simulink model "HeatConductionThroughIronRodSegmented"  (R2024b)
settings: Solver=VariableStepAuto  StartTime=0.0  StopTime=2500  MaxStep=100  RelTol=1e-3  AbsTol=1e-3  EnableMultiTasking=on
PreLoadFcn:
  | if ~exist('D', 'var')            D= 0.025;         end % [m]
  | if ~exist('L', 'var')            L= 0.2;           end % [m]
  | if ~exist('A', 'var')            A= pi*D^2/4;      end % [m^2]
  | if ~exist('A_cyl', 'var')        A_cyl= pi*D*L;    end % [m^2]
  | if ~exist('k', 'var')            k= 80.2;          end % [W/(K*m)]
  | if ~exist('h', 'var')            h= 32.1;          end % [W/(K*m)]
  | if ~exist('m', 'var')            m= 7800*A*L;      end % [kg]
  | if ~exist('c', 'var')            c= 447;           end % [J/kg/K]
  | if ~exist('T_air', 'var')        T_air= 20;        end % [degC]
  | if ~exist('T_base', 'var')       T_base= 100;      end % [degC]
  | if ~exist('T_init', 'var')       T_init= 20;       end % [degC]
  | if ~exist('num_segments', 'var') num_segments= 9; end % [degC]
undefined symbols (not defined in the file): A_cyl, L, m, num_segments, T_init
libraries: fl_lib x45, nesl_utility x7
Description:
  | Heat Conduction Through Iron Rod Using Segmented Model
settings Model: Creator=The MathWorks, Inc.  LastModifiedBy=The MathWorks, Inc.
settings SolverCC: AutoScaleAbsTol=off  AlgebraicLoopSolver=TrustRegion
settings DataIOCC: LimitDataPoints=on  SaveFormat=Array  ReturnWorkspaceOutputs=off  TimeSaveName=tout_segmented_mass_model  OutputSaveName=yout_segmented_mass_model
settings OptimizationCC: LifeSpan=inf
settings DebuggingCC: SolverPrmCheckMsg=warning  UnconnectedInputMsg=warning  UnconnectedOutputMsg=warning  UnconnectedLineMsg=warning  AllowSymbolicDim=off  PregeneratedLibrarySubsystemCodeDiagnostic=none  SFUnexpectedBacktrackingDiag=warning  SFNoUnconditionalDefaultTransitionDiag=warning  SFExecutionAtInitializationDiag=none  ArithmeticOperatorsInVariantConditions=warning
settings HardwareCC: ProdBitPerPointer=32  ProdBitPerSizeT=32  ProdBitPerPtrDiffT=32  ProdLargestAtomicFloat=None  ProdIntDivRoundTo=Undefined  ProdEndianess=Unspecified  ProdWordSize=32  ProdHWDeviceType=32-bit Generic
settings ModelReferenceCC: EnableRefExpFcnMdlSchedulingChecks=on  PropagateSignalLabelsOutOfModel=off
settings SFSimCC: SimUseLocalCustomCode=off  CustomCodeUndefinedFunction=UseInterfaceOnly
settings RTWCC: RTWUseLocalCustomCode=off  GPUComputeCapability=3.5  DLArmComputeVersion=19.05
settings CodeAppCC: StateflowObjectComments=on
settings GRTTargetCC: TargetLangStandard=C89/C90 (ANSI)
settings ConfigComp: CovMetricSettings=dw  CovSaveCumulativeToWorkspaceVar=on  CovSaveSingleToWorkspaceVar=on  CovExternalEMLEnable=off  CovSFcnEnable=off
settings SimscapeCC: SimscapeLogType=all  SimscapeLogSimulationStatistics=on  SimscapeLogName=simlog_HeatConductionThroughIronRodSegmented  SimscapeLogDataHistory=10000

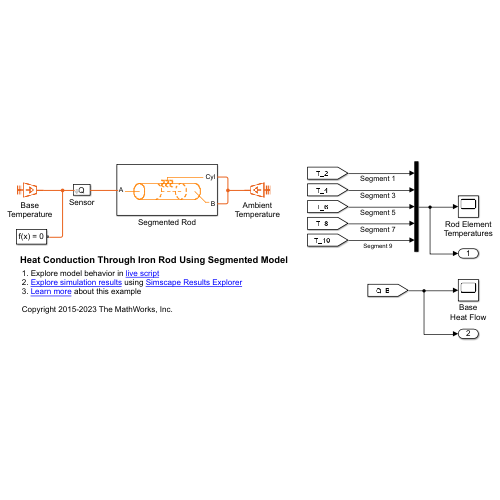
[thumbnail: Simulink's stored preview of the top-level diagram]
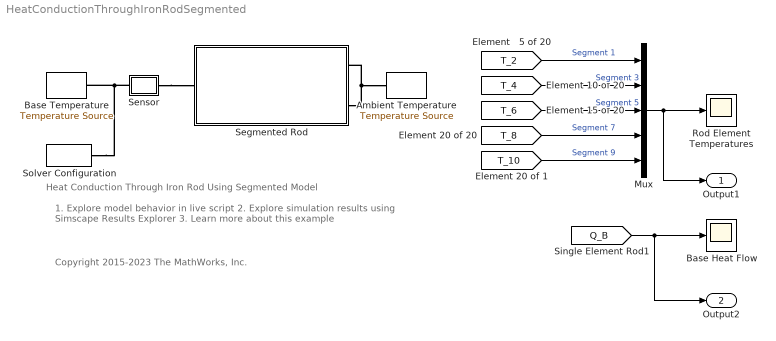
== system HeatConductionThroughIronRodSegmented ==
  note: Heat Conduction Through Iron Rod Using Segmented Model
  note: 1. Explore model behavior in live script
      | 2. Explore simulation results using Simscape Results Explorer
      | 3. Learn more about this example
  note: Copyright 2015-2023 The MathWorks, Inc.
  Ambient Temperature : fl_lib/Thermal/Thermal Sources/Temperature Source  temperature=T_air degC
  Base Heat Flow : Scope
  Base Temperature : fl_lib/Thermal/Thermal Sources/Temperature Source  temperature=T_base degC
  Mux : Mux  Inputs=5
  Rod Element Temperatures : Scope
  Segmented Rod : Subsystem  Tag=PublishSubsystem
      mask Display:
      | color('orange');
      | 
      | % Plot cylinder
      | plot([1,3],[1,1])
      | plot([1,3],[2,2])
      | plot(0.2*cos(0:2*pi/500:2*pi)+1,0.5*sin(0:2*pi/500:2*pi)+1.5)
      | plot(0.2*cos(-pi/2:2*pi/500:pi/2)+3,0.5*sin(-pi/2:2*pi/500:pi/2)+1.5)
      | 
      | % Plot Segmentation
      | plot(0.2*cos(0:2*pi/500:2*pi/16)+2.5,0.5*sin(0:2*pi/500:2*pi/16)+1.5)
      | plot(0.2*cos(2*2*pi/16:2*pi/500:3*2*pi/16)+2.5,0.5*sin(2*2*pi/16:2*pi/500:3*2*pi/16)+1.5)
      | plot(0.2*cos(4*2*pi/16:2*pi/500:5*2*pi/16)+2.5,0.5*sin(4*2*pi/16:2*pi/500:5*2*pi/16)+1.5)
      | plot(0.2*cos(6*2*pi/16:2*pi/500:7*2*pi/16)+2.5,0.5*sin(6*2*pi/16:2*pi/500:7*2*pi/16)+1.5)
      | plot(0.2*cos(8*2*pi/16:2*pi/500:9*2*pi/16)+2.5,0.5*sin(8*2*pi/16:2*pi/500:9*2*pi/16)+1.5)
      | plot(0.2*cos(10*2*pi/16:2*pi/500:11*2*pi/16)+2.5,0.5*sin(10*2*pi/16:2*pi/500:11*2*pi/16)+1.5)
      | plot(0.2*cos(12*2*pi/16:2*pi/500:13*2*pi/16)+2.5,0.5*sin(12*2*pi/16:2*pi/500:13*2*pi/16)+1.5)
      | plot(0.2*cos(14*2*pi/16:2*pi/500:15*2*pi/16)+2.5,0.5*sin(14*2*pi/16:2*pi/500:15*2*pi/16)+1.5)
      | 
      | plot(0.2*cos(0:2*pi/500:2*pi/16)+1.6,0.5*sin(0:2*pi/500:2*pi/16)+1.5)
      | plot(0.2*cos(2*2*pi/16:2*pi/500:3*2*pi/16)+1.6,0.5*sin(2*2*pi/16:2*pi/500:3*2*pi/16)+1.5)
      | plot(0.2*cos(12*2*pi/16:2*pi/500:13*2*pi/16)+1.6,0.5*sin(12*2*pi/16:2*pi/500:13*2*pi/16)+1.5)
      | plot(0.2*cos(14*2*pi/16:2*pi/500:15*2*pi/16)+1.6,0.5*sin(14*2*pi/16:2*pi/500:15*2*pi/16)+1.5)
      | 
      | plot([1.8 1.9],[1.5 1.5])
      | plot([2 2.1],[1.5 1.5])
      | plot([2.2 2.3],[1.5 1.5])
      | plot([2.4 2.5],[1.5 1.5])
      | 
      | % Heat Port
      | plot([1.8 2.2],[2.2 2.2])
      | plot([0.1*cos(-pi/2:0.1:pi/2)+1.8],[0.1*sin(-pi/2:0.1:pi/2)+2.1])
      | plot([0.1*cos(pi/2:0.1:3*pi/2)+1.9],[0.1*sin(pi/2:0.1:3*pi/2)+1.9])
      | plot([0.1*cos(-pi/2:0.1:pi/2)+1.95],[0.1*sin(-pi/2:0.1:pi/2)+2.1])
      | plot([0.1*cos(pi/2:0.1:3*pi/2)+2.05],[0.1*sin(pi/2:0.1:3*pi/2)+1.9])
      | plot([0.1*cos(-pi/2:0.1:pi/2)+2.1],[0.1*sin(-pi/2:0.1:pi/2)+2.1])
      | plot([0.1*cos(pi/2:0.1:3*pi/2)+2.2],[0.1*sin(pi/2:0.1:3*pi/2)+1.9])
      | 
      | % Connecting lines
      | plot([2 3.3],[2.4,2.4])
      | plot([2 2],[2.2 2.4])
      | plot([0.5 1],[1.5 1.5])
      | plot([3.4 3.5],[0.8 0.8])
      | plot([3,3.4],[1.5 0.8])
      | % Scaling
      | color('white')
      | plot(0.2,0)
      | plot(3.8,3.2)
  Sensor : Subsystem
      mask Display: fprintf('Q')
  Solver Configuration : nesl_utility/Solver Configuration  PhysicalDomain=network_engine_domain  SubClassName=solver  LeftPortType=input  RightPortType=generic  Tones=[]  Harmonics=[]  SimulateNoise=off  Profile=off  UseLocalSampling=off  EnableSwitchedLinearOptims=on  FrequencyDomain=off  UseCCode=off  RelTol=0.001  AbsTol=1e-06  MinStep=1e-09  ToWorkspace=off  RevertToSquareIcSolve=off  NumHomotopyIterations=100  PhasorMode=off  PhasorModeNumHarmonics=1  ConsistencySolver=NEWTON_XTOL_AFTER_FTOL  IndexReductionMethod=DerivativeReplacement  DoDC=off  ResidualTolerance=1e-9  ConsistencyTolSource=GLOBAL  ConsistencyAbsTol=0.001  ConsistencyRelTol=0.001  ConsistencyTolFactor=0.001  UseLocalSolver=off  LocalSolverChoice=NE_BACKWARD_EULER_ADVANCER  ResolveIndetEquations=on  FunctionEvalNumThread=1  LocalSolverSampleTime=.001  DoFixedCost=off  MaxNonlinIter=3  MaxModeIter=2  ComputeImpulses=off  ImpulseIterations=2  LinearAlgebra=auto  LinearAlgebraNumThread=0  EquationFormulation=NE_TIME_EF  DelaysMemoryBudget=1024  AutomaticFiltering=on  FilteringTimeConstant=0.001  PartitionStorageMethod=AS_NEEDED  PartitionMemoryBudget=1024  PartitionMethod=FAST  MultibodyUseLocalSolver=off  MultibodyLocalSolverChoice=ODE1  MultibodyLocalSolverSampleTime=0.001
  Output1 : Outport
  Output2 : Outport  Port=2
  wires:
  Mux/1 -> Rod Element Temperatures/1, Output1/1
  [T_6] -> Mux/3  "Segment 5"
  [T_2] -> Mux/1  "Segment 1"
  [T_4] -> Mux/2  "Segment 3"
  [T_8] -> Mux/4  "Segment 7"
  [Q_B] -> Output2/1, Base Heat Flow/1
  [T_10] -> Mux/5  "Segment 9"
  connections:
  Segmented Rod/RConn2 -- Ambient Temperature/LConn1 -- Segmented Rod/RConn1
  Sensor/LConn1 -- Solver Configuration/RConn1 -- Base Temperature/LConn1
  Sensor/RConn1 -- Segmented Rod/LConn1

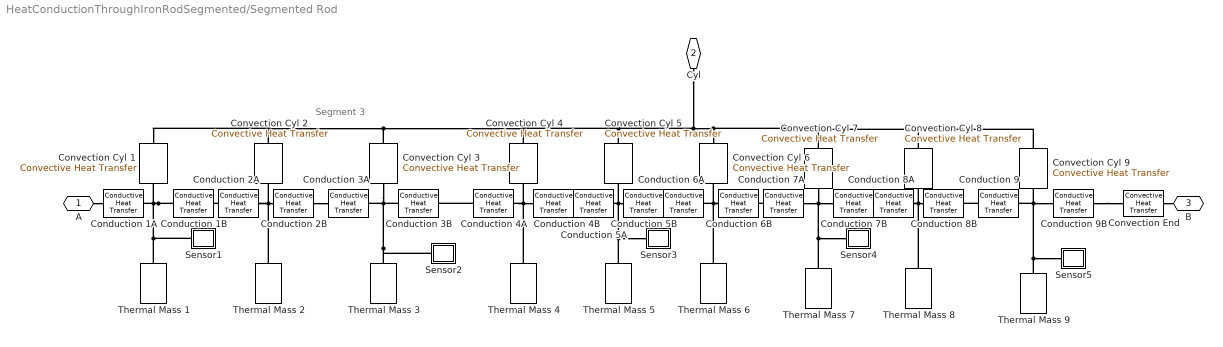
== system HeatConductionThroughIronRodSegmented/Segmented Rod ==
  note: Segment 3
  Conduction 1A : fl_lib/Thermal/Thermal Elements/Conductive Heat Transfer  thermal_type=foundation.enum.ConstantVariableTabulated.Constant  wall_geometry=foundation.enum.ConductionWallGeometry.Planar  area=A m^2  thickness=L/(2*num_segments) m  d_in=0.05 m  d_out=0.1 m  L=1 m  th_cond_min=10 W/(K*m)  th_cond=k W/m/K  th_cond_TLU=[413, 401, 392, 383, 371, 357, 342] W/(K*m)  temp_TLU=[200, 273, 400, 600, 800, 1000, 1200] K  T_specify=off  T_priority=High  T=0 K  T_nominal_specify=off  T_nominal_value=1  T_nominal_unit=K  Q_specify=off  Q_priority=High  Q=0 J/s  Q_nominal_specify=off  Q_nominal_value=1  Q_nominal_unit=J/s
  Conduction 1B : fl_lib/Thermal/Thermal Elements/Conductive Heat Transfer  thermal_type=foundation.enum.ConstantVariableTabulated.Constant  wall_geometry=foundation.enum.ConductionWallGeometry.Planar  area=A m^2  thickness=L/(2*num_segments) m  d_in=0.05 m  d_out=0.1 m  L=1 m  th_cond_min=10 W/(K*m)  th_cond=k W/m/K  th_cond_TLU=[413, 401, 392, 383, 371, 357, 342] W/(K*m)  temp_TLU=[200, 273, 400, 600, 800, 1000, 1200] K  T_specify=off  T_priority=High  T=0 K  T_nominal_specify=off  T_nominal_value=1  T_nominal_unit=K  Q_specify=off  Q_priority=High  Q=0 J/s  Q_nominal_specify=off  Q_nominal_value=1  Q_nominal_unit=J/s
  Conduction 2A : fl_lib/Thermal/Thermal Elements/Conductive Heat Transfer  thermal_type=foundation.enum.ConstantVariableTabulated.Constant  wall_geometry=foundation.enum.ConductionWallGeometry.Planar  area=A m^2  thickness=L/(2*num_segments) m  d_in=0.05 m  d_out=0.1 m  L=1 m  th_cond_min=10 W/(K*m)  th_cond=k W/m/K  th_cond_TLU=[413, 401, 392, 383, 371, 357, 342] W/(K*m)  temp_TLU=[200, 273, 400, 600, 800, 1000, 1200] K  T_specify=off  T_priority=High  T=0 K  T_nominal_specify=off  T_nominal_value=1  T_nominal_unit=K  Q_specify=off  Q_priority=High  Q=0 J/s  Q_nominal_specify=off  Q_nominal_value=1  Q_nominal_unit=J/s
  Conduction 2B : fl_lib/Thermal/Thermal Elements/Conductive Heat Transfer  thermal_type=foundation.enum.ConstantVariableTabulated.Constant  wall_geometry=foundation.enum.ConductionWallGeometry.Planar  area=A m^2  thickness=L/(2*num_segments) m  d_in=0.05 m  d_out=0.1 m  L=1 m  th_cond_min=10 W/(K*m)  th_cond=k W/m/K  th_cond_TLU=[413, 401, 392, 383, 371, 357, 342] W/(K*m)  temp_TLU=[200, 273, 400, 600, 800, 1000, 1200] K  T_specify=off  T_priority=High  T=0 K  T_nominal_specify=off  T_nominal_value=1  T_nominal_unit=K  Q_specify=off  Q_priority=High  Q=0 J/s  Q_nominal_specify=off  Q_nominal_value=1  Q_nominal_unit=J/s
  Conduction 3A : fl_lib/Thermal/Thermal Elements/Conductive Heat Transfer  thermal_type=foundation.enum.ConstantVariableTabulated.Constant  wall_geometry=foundation.enum.ConductionWallGeometry.Planar  area=A m^2  thickness=L/(2*num_segments) m  d_in=0.05 m  d_out=0.1 m  L=1 m  th_cond_min=10 W/(K*m)  th_cond=k W/m/K  th_cond_TLU=[413, 401, 392, 383, 371, 357, 342] W/(K*m)  temp_TLU=[200, 273, 400, 600, 800, 1000, 1200] K  T_specify=off  T_priority=High  T=0 K  T_nominal_specify=off  T_nominal_value=1  T_nominal_unit=K  Q_specify=off  Q_priority=High  Q=0 J/s  Q_nominal_specify=off  Q_nominal_value=1  Q_nominal_unit=J/s
  Conduction 3B : fl_lib/Thermal/Thermal Elements/Conductive Heat Transfer  thermal_type=foundation.enum.ConstantVariableTabulated.Constant  wall_geometry=foundation.enum.ConductionWallGeometry.Planar  area=A m^2  thickness=L/(2*num_segments) m  d_in=0.05 m  d_out=0.1 m  L=1 m  th_cond_min=10 W/(K*m)  th_cond=k W/m/K  th_cond_TLU=[413, 401, 392, 383, 371, 357, 342] W/(K*m)  temp_TLU=[200, 273, 400, 600, 800, 1000, 1200] K  T_specify=off  T_priority=High  T=0 K  T_nominal_specify=off  T_nominal_value=1  T_nominal_unit=K  Q_specify=off  Q_priority=High  Q=0 J/s  Q_nominal_specify=off  Q_nominal_value=1  Q_nominal_unit=J/s
  Conduction 4A : fl_lib/Thermal/Thermal Elements/Conductive Heat Transfer  thermal_type=foundation.enum.ConstantVariableTabulated.Constant  wall_geometry=foundation.enum.ConductionWallGeometry.Planar  area=A m^2  thickness=L/(2*num_segments) m  d_in=0.05 m  d_out=0.1 m  L=1 m  th_cond_min=10 W/(K*m)  th_cond=k W/m/K  th_cond_TLU=[413, 401, 392, 383, 371, 357, 342] W/(K*m)  temp_TLU=[200, 273, 400, 600, 800, 1000, 1200] K  T_specify=off  T_priority=High  T=0 K  T_nominal_specify=off  T_nominal_value=1  T_nominal_unit=K  Q_specify=off  Q_priority=High  Q=0 J/s  Q_nominal_specify=off  Q_nominal_value=1  Q_nominal_unit=J/s
  Conduction 4B : fl_lib/Thermal/Thermal Elements/Conductive Heat Transfer  thermal_type=foundation.enum.ConstantVariableTabulated.Constant  wall_geometry=foundation.enum.ConductionWallGeometry.Planar  area=A m^2  thickness=L/(2*num_segments) m  d_in=0.05 m  d_out=0.1 m  L=1 m  th_cond_min=10 W/(K*m)  th_cond=k W/m/K  th_cond_TLU=[413, 401, 392, 383, 371, 357, 342] W/(K*m)  temp_TLU=[200, 273, 400, 600, 800, 1000, 1200] K  T_specify=off  T_priority=High  T=0 K  T_nominal_specify=off  T_nominal_value=1  T_nominal_unit=K  Q_specify=off  Q_priority=High  Q=0 J/s  Q_nominal_specify=off  Q_nominal_value=1  Q_nominal_unit=J/s
  Conduction 5A : fl_lib/Thermal/Thermal Elements/Conductive Heat Transfer  thermal_type=foundation.enum.ConstantVariableTabulated.Constant  wall_geometry=foundation.enum.ConductionWallGeometry.Planar  area=A m^2  thickness=L/(2*num_segments) m  d_in=0.05 m  d_out=0.1 m  L=1 m  th_cond_min=10 W/(K*m)  th_cond=k W/m/K  th_cond_TLU=[413, 401, 392, 383, 371, 357, 342] W/(K*m)  temp_TLU=[200, 273, 400, 600, 800, 1000, 1200] K  T_specify=off  T_priority=High  T=0 K  T_nominal_specify=off  T_nominal_value=1  T_nominal_unit=K  Q_specify=off  Q_priority=High  Q=0 J/s  Q_nominal_specify=off  Q_nominal_value=1  Q_nominal_unit=J/s
  Conduction 5B : fl_lib/Thermal/Thermal Elements/Conductive Heat Transfer  thermal_type=foundation.enum.ConstantVariableTabulated.Constant  wall_geometry=foundation.enum.ConductionWallGeometry.Planar  area=A m^2  thickness=L/(2*num_segments) m  d_in=0.05 m  d_out=0.1 m  L=1 m  th_cond_min=10 W/(K*m)  th_cond=k W/m/K  th_cond_TLU=[413, 401, 392, 383, 371, 357, 342] W/(K*m)  temp_TLU=[200, 273, 400, 600, 800, 1000, 1200] K  T_specify=off  T_priority=High  T=0 K  T_nominal_specify=off  T_nominal_value=1  T_nominal_unit=K  Q_specify=off  Q_priority=High  Q=0 J/s  Q_nominal_specify=off  Q_nominal_value=1  Q_nominal_unit=J/s
  Conduction 6A : fl_lib/Thermal/Thermal Elements/Conductive Heat Transfer  thermal_type=foundation.enum.ConstantVariableTabulated.Constant  wall_geometry=foundation.enum.ConductionWallGeometry.Planar  area=A m^2  thickness=L/(2*num_segments) m  d_in=0.05 m  d_out=0.1 m  L=1 m  th_cond_min=10 W/(K*m)  th_cond=k W/m/K  th_cond_TLU=[413, 401, 392, 383, 371, 357, 342] W/(K*m)  temp_TLU=[200, 273, 400, 600, 800, 1000, 1200] K  T_specify=off  T_priority=High  T=0 K  T_nominal_specify=off  T_nominal_value=1  T_nominal_unit=K  Q_specify=off  Q_priority=High  Q=0 J/s  Q_nominal_specify=off  Q_nominal_value=1  Q_nominal_unit=J/s
  Conduction 6B : fl_lib/Thermal/Thermal Elements/Conductive Heat Transfer  thermal_type=foundation.enum.ConstantVariableTabulated.Constant  wall_geometry=foundation.enum.ConductionWallGeometry.Planar  area=A m^2  thickness=L/(2*num_segments) m  d_in=0.05 m  d_out=0.1 m  L=1 m  th_cond_min=10 W/(K*m)  th_cond=k W/m/K  th_cond_TLU=[413, 401, 392, 383, 371, 357, 342] W/(K*m)  temp_TLU=[200, 273, 400, 600, 800, 1000, 1200] K  T_specify=off  T_priority=High  T=0 K  T_nominal_specify=off  T_nominal_value=1  T_nominal_unit=K  Q_specify=off  Q_priority=High  Q=0 J/s  Q_nominal_specify=off  Q_nominal_value=1  Q_nominal_unit=J/s
  Conduction 7A : fl_lib/Thermal/Thermal Elements/Conductive Heat Transfer  thermal_type=foundation.enum.ConstantVariableTabulated.Constant  wall_geometry=foundation.enum.ConductionWallGeometry.Planar  area=A m^2  thickness=L/(2*num_segments) m  d_in=0.05 m  d_out=0.1 m  L=1 m  th_cond_min=10 W/(K*m)  th_cond=k W/m/K  th_cond_TLU=[413, 401, 392, 383, 371, 357, 342] W/(K*m)  temp_TLU=[200, 273, 400, 600, 800, 1000, 1200] K  T_specify=off  T_priority=High  T=0 K  T_nominal_specify=off  T_nominal_value=1  T_nominal_unit=K  Q_specify=off  Q_priority=High  Q=0 J/s  Q_nominal_specify=off  Q_nominal_value=1  Q_nominal_unit=J/s
  Conduction 7B : fl_lib/Thermal/Thermal Elements/Conductive Heat Transfer  thermal_type=foundation.enum.ConstantVariableTabulated.Constant  wall_geometry=foundation.enum.ConductionWallGeometry.Planar  area=A m^2  thickness=L/(2*num_segments) m  d_in=0.05 m  d_out=0.1 m  L=1 m  th_cond_min=10 W/(K*m)  th_cond=k W/m/K  th_cond_TLU=[413, 401, 392, 383, 371, 357, 342] W/(K*m)  temp_TLU=[200, 273, 400, 600, 800, 1000, 1200] K  T_specify=off  T_priority=High  T=0 K  T_nominal_specify=off  T_nominal_value=1  T_nominal_unit=K  Q_specify=off  Q_priority=High  Q=0 J/s  Q_nominal_specify=off  Q_nominal_value=1  Q_nominal_unit=J/s
  Conduction 8A : fl_lib/Thermal/Thermal Elements/Conductive Heat Transfer  thermal_type=foundation.enum.ConstantVariableTabulated.Constant  wall_geometry=foundation.enum.ConductionWallGeometry.Planar  area=A m^2  thickness=L/(2*num_segments) m  d_in=0.05 m  d_out=0.1 m  L=1 m  th_cond_min=10 W/(K*m)  th_cond=k W/m/K  th_cond_TLU=[413, 401, 392, 383, 371, 357, 342] W/(K*m)  temp_TLU=[200, 273, 400, 600, 800, 1000, 1200] K  T_specify=off  T_priority=High  T=0 K  T_nominal_specify=off  T_nominal_value=1  T_nominal_unit=K  Q_specify=off  Q_priority=High  Q=0 J/s  Q_nominal_specify=off  Q_nominal_value=1  Q_nominal_unit=J/s
  Conduction 8B : fl_lib/Thermal/Thermal Elements/Conductive Heat Transfer  thermal_type=foundation.enum.ConstantVariableTabulated.Constant  wall_geometry=foundation.enum.ConductionWallGeometry.Planar  area=A m^2  thickness=L/(2*num_segments) m  d_in=0.05 m  d_out=0.1 m  L=1 m  th_cond_min=10 W/(K*m)  th_cond=k W/m/K  th_cond_TLU=[413, 401, 392, 383, 371, 357, 342] W/(K*m)  temp_TLU=[200, 273, 400, 600, 800, 1000, 1200] K  T_specify=off  T_priority=High  T=0 K  T_nominal_specify=off  T_nominal_value=1  T_nominal_unit=K  Q_specify=off  Q_priority=High  Q=0 J/s  Q_nominal_specify=off  Q_nominal_value=1  Q_nominal_unit=J/s
  Conduction 9 : fl_lib/Thermal/Thermal Elements/Conductive Heat Transfer  thermal_type=foundation.enum.ConstantVariableTabulated.Constant  wall_geometry=foundation.enum.ConductionWallGeometry.Planar  area=A m^2  thickness=L/(2*num_segments) m  d_in=0.05 m  d_out=0.1 m  L=1 m  th_cond_min=10 W/(K*m)  th_cond=k W/m/K  th_cond_TLU=[413, 401, 392, 383, 371, 357, 342] W/(K*m)  temp_TLU=[200, 273, 400, 600, 800, 1000, 1200] K  T_specify=off  T_priority=High  T=0 K  T_nominal_specify=off  T_nominal_value=1  T_nominal_unit=K  Q_specify=off  Q_priority=High  Q=0 J/s  Q_nominal_specify=off  Q_nominal_value=1  Q_nominal_unit=J/s
  Conduction 9B : fl_lib/Thermal/Thermal Elements/Conductive Heat Transfer  thermal_type=foundation.enum.ConstantVariableTabulated.Constant  wall_geometry=foundation.enum.ConductionWallGeometry.Planar  area=A m^2  thickness=L/(2*num_segments) m  d_in=0.05 m  d_out=0.1 m  L=1 m  th_cond_min=10 W/(K*m)  th_cond=k W/m/K  th_cond_TLU=[413, 401, 392, 383, 371, 357, 342] W/(K*m)  temp_TLU=[200, 273, 400, 600, 800, 1000, 1200] K  T_specify=off  T_priority=High  T=0 K  T_nominal_specify=off  T_nominal_value=1  T_nominal_unit=K  Q_specify=off  Q_priority=High  Q=0 J/s  Q_nominal_specify=off  Q_nominal_value=1  Q_nominal_unit=J/s
  Convection Cyl {1..9} (9 alike) : fl_lib/Thermal/Thermal Elements/Convective Heat Transfer  thermal_type=foundation.enum.constant_variable.constant  area=A_cyl/num_segments m^2  heat_tr_coeff=h W/m^2/K  min_heat_tr_coeff=1e-3 W/(K*m^2)  T_specify=off  T_priority=High  T=0 K  T_nominal_specify=off  T_nominal_value=1  T_nominal_unit=K  Q_specify=off  Q_priority=High  Q=0 J/s  Q_nominal_specify=off  Q_nominal_value=1  Q_nominal_unit=J/s
  Convection End : fl_lib/Thermal/Thermal Elements/Convective Heat Transfer  thermal_type=foundation.enum.constant_variable.constant  area=A m^2  heat_tr_coeff=h W/(m^2 * K)  min_heat_tr_coeff=1e-3 W/(K*m^2)  T_specify=off  T_priority=None  T=0 K  T_nominal_specify=off  T_nominal_value=1  T_nominal_unit=K  Q_specify=off  Q_priority=None  Q=0 W  Q_nominal_specify=off  Q_nominal_value=1  Q_nominal_unit=W
  Sensor1 : Subsystem
      mask Display: disp('T')
  Sensor2 : Subsystem
      mask Display: disp('T')
  Sensor3 : Subsystem
      mask Display: disp('T')
  Sensor4 : Subsystem
      mask Display: disp('T')
  Sensor5 : Subsystem
      mask Display: disp('T')
  Thermal Mass {1..9} (9 alike) : fl_lib/Thermal/Thermal Elements/Thermal Mass  mass_type=foundation.enum.constant_variable.constant  mass=m/num_segments kg  sp_heat=c J/kg/K  mass_min=1e-6 kg  num_ports=foundation.enum.numPorts2.one  m_specify=off  m_priority=High  m=1 kg  m_nominal_specify=off  m_nominal_value=1  m_nominal_unit=kg  T_specify=on  T_priority=High  T=T_init degC  T_nominal_specify=off  T_nominal_value=1  T_nominal_unit=K  Q_specify=off  Q_priority=None  Q=0 W  Q_nominal_specify=off  Q_nominal_value=1  Q_nominal_unit=W
  A : PMIOPort  Side=Left
  Cyl : PMIOPort  Port=2  Side=Right
  B : PMIOPort  Port=3  Side=Right
  connections:
  Conduction 5A/LConn1 -- Conduction 4B/RConn1
  Conduction 2B/RConn1 -- Conduction 3A/LConn1
  A/RConn1 -- Conduction 1A/LConn1
  Conduction 2A/LConn1 -- Conduction 1B/RConn1
  Conduction 4A/LConn1 -- Conduction 3B/RConn1
  Convection Cyl 5/LConn1 -- Thermal Mass 5/LConn1 -- Sensor3/LConn1 -- Conduction 5A/RConn1 -- Conduction 5B/LConn1
  Conduction 4B/LConn1 -- Thermal Mass 4/LConn1 -- Convection Cyl 4/LConn1 -- Conduction 4A/RConn1
  Thermal Mass 3/LConn1 -- Sensor2/LConn1 -- Conduction 3B/LConn1 -- Convection Cyl 3/LConn1 -- Conduction 3A/RConn1
  Conduction 2B/LConn1 -- Thermal Mass 2/LConn1 -- Conduction 2A/RConn1 -- Convection Cyl 2/LConn1
  Thermal Mass 1/LConn1 -- Sensor1/LConn1 -- Conduction 1B/LConn1 -- Conduction 1A/RConn1 -- Convection Cyl 1/LConn1
  Conduction 7B/RConn1 -- Conduction 8A/LConn1
  Conduction 5B/RConn1 -- Conduction 6A/LConn1
  Conduction 7A/LConn1 -- Conduction 6B/RConn1
  Conduction 6A/RConn1 -- Thermal Mass 6/LConn1 -- Convection Cyl 6/LConn1 -- Conduction 6B/LConn1
  Cyl/RConn1 -- Convection Cyl 5/RConn1 -- Convection Cyl 2/RConn1 -- Convection Cyl 1/RConn1 -- Convection Cyl 3/RConn1 -- Convection Cyl 4/RConn1 -- Convection Cyl 9/RConn1 -- Convection Cyl 8/RConn1 -- Convection Cyl 7/RConn1 -- Convection Cyl 6/RConn1
  Conduction 7A/RConn1 -- Sensor4/LConn1 -- Thermal Mass 7/LConn1 -- Conduction 7B/LConn1 -- Convection Cyl 7/LConn1
  Conduction 8B/LConn1 -- Thermal Mass 8/LConn1 -- Convection Cyl 8/LConn1 -- Conduction 8A/RConn1
  Conduction 9/RConn1 -- Thermal Mass 9/LConn1 -- Sensor5/LConn1 -- Convection Cyl 9/LConn1 -- Conduction 9B/LConn1
  Conduction 9/LConn1 -- Conduction 8B/RConn1
  Conduction 9B/RConn1 -- Convection End/LConn1
  Convection End/RConn1 -- B/RConn1

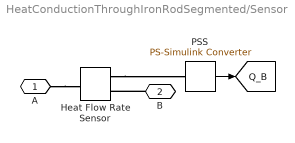
== system HeatConductionThroughIronRodSegmented/Sensor ==
  Heat Flow Rate Sensor : fl_lib/Thermal/Thermal Sensors/Heat Flow Rate Sensor
  PSS : nesl_utility/PS-Simulink Converter  PhysicalDomain=network_engine_domain  SubClassName=ps_output  LeftPortType=input  RightPortType=output  PseudoPeriodic=off  Frequencies=[]  VectorFormat=1-D array  Unit=W  AffineConversion=off
  A : PMIOPort  Side=Left
  B : PMIOPort  Port=2  Side=Right
  tag scope: Q_B=global
  wires:
  PSS/1 -> [Q_B]
  connections:
  A/RConn1 -- Heat Flow Rate Sensor/LConn1
  B/RConn1 -- Heat Flow Rate Sensor/RConn2
  Heat Flow Rate Sensor/RConn1 -- PSS/LConn1

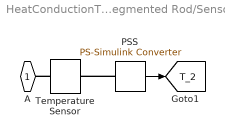
== system HeatConductionThroughIronRodSegmented/Segmented Rod/Sensor1 ==
  PSS : nesl_utility/PS-Simulink Converter  PhysicalDomain=network_engine_domain  SubClassName=ps_output  LeftPortType=input  RightPortType=output  PseudoPeriodic=off  Frequencies=[]  VectorFormat=1-D array  Unit=degC  AffineConversion=on
  Temperature Sensor : fl_lib/Thermal/Thermal Sensors/Temperature Sensor  temperature_measure=foundation.enum.MeasurementReference.absolute
      settings: InternalSimscapePortConfiguration="{\"Bottom\":[],\"Left\":[{\"id\":\"A\",\"label\":\"A\",\"type\":\"foundation.thermal.thermal\"}],\"Right\":[{\"id\":\"T\",\"label\":\"T\",\"type\":\"output\"}],\"Top\":[]}"
  A : PMIOPort  Side=Left
  tag scope: T_2=global
  wires:
  PSS/1 -> [T_2]
  connections:
  PSS/LConn1 -- Temperature Sensor/RConn1
  Temperature Sensor/LConn1 -- A/RConn1

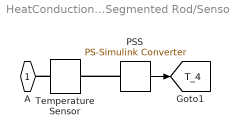
== system HeatConductionThroughIronRodSegmented/Segmented Rod/Sensor2 ==
  PSS : nesl_utility/PS-Simulink Converter  PhysicalDomain=network_engine_domain  SubClassName=ps_output  LeftPortType=input  RightPortType=output  PseudoPeriodic=off  Frequencies=[]  VectorFormat=1-D array  Unit=degC  AffineConversion=on
  Temperature Sensor : fl_lib/Thermal/Thermal Sensors/Temperature Sensor  temperature_measure=foundation.enum.MeasurementReference.absolute
      settings: InternalSimscapePortConfiguration="{\"Bottom\":[],\"Left\":[{\"id\":\"A\",\"label\":\"A\",\"type\":\"foundation.thermal.thermal\"}],\"Right\":[{\"id\":\"T\",\"label\":\"T\",\"type\":\"output\"}],\"Top\":[]}"
  A : PMIOPort  Side=Left
  tag scope: T_4=global
  wires:
  PSS/1 -> [T_4]
  connections:
  PSS/LConn1 -- Temperature Sensor/RConn1
  Temperature Sensor/LConn1 -- A/RConn1

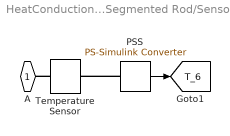
== system HeatConductionThroughIronRodSegmented/Segmented Rod/Sensor3 ==
  PSS : nesl_utility/PS-Simulink Converter  PhysicalDomain=network_engine_domain  SubClassName=ps_output  LeftPortType=input  RightPortType=output  PseudoPeriodic=off  Frequencies=[]  VectorFormat=1-D array  Unit=degC  AffineConversion=on
  Temperature Sensor : fl_lib/Thermal/Thermal Sensors/Temperature Sensor  temperature_measure=foundation.enum.MeasurementReference.absolute
      settings: InternalSimscapePortConfiguration="{\"Bottom\":[],\"Left\":[{\"id\":\"A\",\"label\":\"A\",\"type\":\"foundation.thermal.thermal\"}],\"Right\":[{\"id\":\"T\",\"label\":\"T\",\"type\":\"output\"}],\"Top\":[]}"
  A : PMIOPort  Side=Left
  tag scope: T_6=global
  wires:
  PSS/1 -> [T_6]
  connections:
  PSS/LConn1 -- Temperature Sensor/RConn1
  Temperature Sensor/LConn1 -- A/RConn1

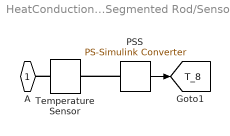
== system HeatConductionThroughIronRodSegmented/Segmented Rod/Sensor4 ==
  PSS : nesl_utility/PS-Simulink Converter  PhysicalDomain=network_engine_domain  SubClassName=ps_output  LeftPortType=input  RightPortType=output  PseudoPeriodic=off  Frequencies=[]  VectorFormat=1-D array  Unit=degC  AffineConversion=on
  Temperature Sensor : fl_lib/Thermal/Thermal Sensors/Temperature Sensor  temperature_measure=foundation.enum.MeasurementReference.absolute
      settings: InternalSimscapePortConfiguration="{\"Bottom\":[],\"Left\":[{\"id\":\"A\",\"label\":\"A\",\"type\":\"foundation.thermal.thermal\"}],\"Right\":[{\"id\":\"T\",\"label\":\"T\",\"type\":\"output\"}],\"Top\":[]}"
  A : PMIOPort  Side=Left
  tag scope: T_8=global
  wires:
  PSS/1 -> [T_8]
  connections:
  PSS/LConn1 -- Temperature Sensor/RConn1
  Temperature Sensor/LConn1 -- A/RConn1

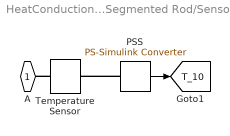
== system HeatConductionThroughIronRodSegmented/Segmented Rod/Sensor5 ==
  PSS : nesl_utility/PS-Simulink Converter  PhysicalDomain=network_engine_domain  SubClassName=ps_output  LeftPortType=input  RightPortType=output  PseudoPeriodic=off  Frequencies=[]  VectorFormat=1-D array  Unit=degC  AffineConversion=on
  Temperature Sensor : fl_lib/Thermal/Thermal Sensors/Temperature Sensor  temperature_measure=foundation.enum.MeasurementReference.absolute
      settings: InternalSimscapePortConfiguration="{\"Bottom\":[],\"Left\":[{\"id\":\"A\",\"label\":\"A\",\"type\":\"foundation.thermal.thermal\"}],\"Right\":[{\"id\":\"T\",\"label\":\"T\",\"type\":\"output\"}],\"Top\":[]}"
  A : PMIOPort  Side=Left
  tag scope: T_10=global
  wires:
  PSS/1 -> [T_10]
  connections:
  PSS/LConn1 -- Temperature Sensor/RConn1
  Temperature Sensor/LConn1 -- A/RConn1
